simulink model "mcb_pmsm_foc_sensorless_f28379d"  (R2023b)
settings: Solver=FixedStepDiscrete  StartTime=0.0  StopTime=6  FixedStep=Auto  RelTol=1e-3  EnableMultiTasking=on
InitFcn:
  | mcb_pmsm_foc_sensorless_f28379d_datascript;
model workspace (MAT data in the model file):
  encoderResolution = 2000
  hallOffset = '0.5'
  indexOffset = 850
  polePairs = '4'
values from neighbouring files (symbols this model uses):
  acceleration = 0.5/Ts_speed/PU_System.N_base    [mcb_pmsm_foc_sensorless_f28379d_datascript.m]
  dataType = 'single'    [mcb_pmsm_foc_sensorless_f28379d_datascript.m]    (also in mcb_pmsm_foc_test_f28379d_data.m)
  inverter = mcb_updateInverterParameters(pmsm,inverter,target)    [mcb_pmsm_foc_sensorless_f28379d_datascript.m]    (also in mcb_pmsm_foc_test_f28379d_data.m)
  PI_params = mcb_SetControllerParameters(pmsm,inverter,PU_System,T_pwm,2*Ts,Ts_speed)    [mcb_pmsm_foc_sensorless_f28379d_datascript.m]    (also in mcb_pmsm_foc_test_f28379d_data.m = mcb_SetControllerParameters(pmsm,inverter,PU_System,T_pwm,Ts)
  pmsm = mcb_SetPMSMMotorParameters("new")    [mcb_pmsm_foc_sensorless_f28379d_datascript.m]    (also in mcb_pmsm_foc_test_f28379d_data.m = mcb_SetPMSMMotorParameters("SF2804"))
  PU_System = mcb_SetPUSystem(pmsm,inverter)    [mcb_pmsm_foc_sensorless_f28379d_datascript.m]    (also in mcb_pmsm_foc_test_f28379d_data.m)
  Speed_openLoop_PU = 0.1    [mcb_pmsm_foc_sensorless_f28379d_datascript.m]
  T = Ts    (= 5e-05)    [mcb_pmsm_foc_sensorless_f28379d_datascript.m]
  T_Ref_openLoop = 1    [mcb_pmsm_foc_sensorless_f28379d_datascript.m]
  target = mcb_SetProcessorDetails('F28379D',PWM_frequency)    [mcb_pmsm_foc_sensorless_f28379d_datascript.m]    (also in mcb_pmsm_foc_test_f28379d_data.m)
  Ts = T_pwm    [discrete_tansfer_fcn.m]    (also in mcb_pmsm_foc_sensorless_f28379d_datascript.m = 5e-05; mcb_pmsm_foc_test_f28379d_data.m = 5e-05)
  Ts_motor = T_pwm/2    (= 2.5e-05)    [mcb_pmsm_foc_sensorless_f28379d_datascript.m]    (also in mcb_pmsm_foc_test_f28379d_data.m)
  Ts_sensor = 20*Ts    (= 0.001)    [mcb_pmsm_foc_sensorless_f28379d_datascript.m]    (also in mcb_pmsm_foc_test_f28379d_data.m; virtual_speed.m)
  Ts_simulink = T_pwm/2    (= 2.5e-05)    [mcb_pmsm_foc_sensorless_f28379d_datascript.m]    (also in mcb_pmsm_foc_test_f28379d_data.m)
  Ts_speed = 20*Ts    (= 0.001)    [mcb_pmsm_foc_sensorless_f28379d_datascript.m]    (also in mcb_pmsm_foc_test_f28379d_data.m = 0.0005)
undefined symbols (not defined in the file or in its folder): DiscIntNeverNeededParam, Down, GPTRIP1SEL, GPTRIP2SEL, TZ1, TZ2, Up
libraries: mcbcontrolslib x13, simulink x12, c2802xlib x7, mcbpositiondecoderlib x5, c280xlib x5, slpidlib x4, c2837xDlib x4, mcbsensorlessestimatorlib x2, svdschedulerlib x2, svdutilitieslib x1, mcbplantlib x1, autolibpmsmexterior x1
(part 3 of 4)

== system mcb_pmsm_foc_sensorless_f28379d/Current Control/Input Scaling/Calculate position and speed/EKF Observer ==
  InputSignals : Inport
  Action Port : ActionPort  ActionPortLabel=case [ 3 ]:
  Cast To Single : DataTypeConversion  OutDataTypeStr=single  SaturateOnIntegerOverflow=off  RndMeth=Floor
  Data Store Read1 : DataStoreRead  DataStoreName=Enable  IndexOptions=Index vector (dialog)  Indices=1  OutputSizes=1
  Demux1 : Demux
  EKF : Subsystem
  Logical Operator : Logic  Operator=NOT  IconShape=distinctive  AllPortsSameDT=off  OutDataTypeStr=boolean
  Mux2 : Mux  Inputs=2
  Position/Speed : Outport
  wires:
  Data Store Read1/1 -> Logical Operator/1
  InputSignals/1 -> Demux1/1
  Demux1/1 -> EKF/1(ualpha)
  Demux1/2 -> EKF/2(ubeta)
  Demux1/3 -> EKF/3(i_alpha)  "Ialpha"
  Demux1/4 -> EKF/4(i_beta)  "Ibeta"
  Mux2/1 -> Cast To Single/1
  Cast To Single/1 -> Position/Speed/1
  Logical Operator/1 -> EKF/5(Rst)
  EKF/1(theta_hat) -> Mux2/1
  EKF/2(omega_hat) -> Mux2/2  "omega_hat"

== system mcb_pmsm_foc_sensorless_f28379d/Current Control/Input Scaling/Calculate position and speed/Extended EMF Observer ==
  InputSignals : Inport
  Action Port : ActionPort  ActionPortLabel=case [ 2 ]:
  Data Store Read1 : DataStoreRead  DataStoreName=Enable  IndexOptions=Index vector (dialog)  Indices=1  OutputSizes=1
  Demux1 : Demux
  Extended EMF Observer : mcbsensorlessestimatorlib/Extended EMF Observer  InputUnit=Per-unit  PosOut=Electrical position  BlkSampleTime=Ts  StatorResistance=pmsm.Rs  StatorDaxisInductance=pmsm.Ld  StatorQaxisInductance=pmsm.Lq  MaxApplicationSpeed=pmsm.N_base  PolePairs=pmsm.p  MaxStatorVoltage=PU_System.V_base  MaxStatorCurrent=PU_System.I_base  Alpha=10  EEMFCutoffFreq=7500  Kp=250  Ki=200000  N_points=1024  SpeedCutoffFreq=15  PositionUnit=Per-unit  PositionDataType=dataType  SpeedUnit=Per-unit  PerUnitSpeed=PU_System.N_base  SpeedDataType=dataType  TableDatatype=single
      settings: LibrarySourceBlock=mcblib/Sensorless Estimators/Extended EMF Observer
  Logical Operator : Logic  Operator=NOT  IconShape=distinctive  AllPortsSameDT=off  OutDataTypeStr=boolean
  Mux2 : Mux  Inputs=2
  Position/Speed : Outport
  wires:
  Mux2/1 -> Position/Speed/1
  Demux1/3 -> Extended EMF Observer/3  "Ialpha"
  Demux1/4 -> Extended EMF Observer/4  "Ibeta"
  Logical Operator/1 -> Extended EMF Observer/5
  Data Store Read1/1 -> Logical Operator/1
  Demux1/1 -> Extended EMF Observer/1
  Demux1/2 -> Extended EMF Observer/2
  InputSignals/1 -> Demux1/1
  Extended EMF Observer/1 -> Mux2/1
  Extended EMF Observer/2 -> Mux2/2

== system mcb_pmsm_foc_sensorless_f28379d/Current Control/Input Scaling/Calculate position and speed/Flux Observer ==
  InputSignals : Inport
  Action Port : ActionPort  ActionPortLabel=case [ 1 ]:
  DC component removal : Subsystem
  Data Store Read1 : DataStoreRead  DataStoreName=Enable  IndexOptions=Index vector (dialog)  Indices=1  OutputSizes=1
  Demux1 : Demux
  Flux Observer : mcbpositiondecoderlib/Flux Observer  MotorSelection=PMSM  DataTypeSelect=off  BlockInputUnit=Per-unit  PerUnitVoltage=PU_System.V_base  PerUnitCurrent=PU_System.I_base  PositionSelect=on  FluxSelect=off  TorqueSelect=off  PolePairs=4  StatorResistance=pmsm.Rs  StatorDAxisInductance=pmsm.Ld  StatorLeakageInductance=0.0068  RotorLeakageInductance=0.0068  MagnetizingInductance=0.0300  CutoffFreq=3.1863  BlockSampleTime=Ts  PositionUnit=Per-unit  PositionDatatype=dataType  FluxUnit=Weber  PerUnitFlux=0.1  FluxDatatype=single  TorqueUnit=Nm  PerUnitTorque=100  TorqueDatatype=single  DataType=0
  IIR Filter4 : mcbcontrolslib/IIR Filter  VariantControl=Low Pass Filter  VariantSelect=Low-pass  Filter_constant=0.01  advancedSettings=off  Ts=50e-6  cutOff_freq=32.1525
  Logical Operator : Logic  Operator=NOT  IconShape=distinctive  AllPortsSameDT=off  OutDataTypeStr=boolean
  Mux2 : Mux  Inputs=2
  Speed Measurement : mcbpositiondecoderlib/Speed Measurement  PositionUnit=Per unit  PositionScalingDatatype=uint32  SpeedCalculationMode=Time interval for speed calculation  SampleTimeAsync=Ts  MaximumApplicationSpeed=60000  SpeedResolution=5e-6  DelayLength=10  MaximumMeasurableSpeed=59999  MeasurableSpeedResolution=2.794e-05  SpeedUnit=Per unit based on dialog  PerUnitSpeed=PU_System.N_base  SpeedDataType=dataType
  elect2mech : Gain  Gain=1/pmsm.p  RndMeth=Simplest  OutDataTypeStr=Inherit: Same as input
  Position/Speed : Outport
  wires:
  InputSignals/1 -> DC component removal/1(SigIN)
  Mux2/1 -> Position/Speed/1
  Speed Measurement/1 -> IIR Filter4/1
  elect2mech/1 -> Mux2/2
  Demux1/3 -> Flux Observer/3  "Ialpha"
  Demux1/4 -> Flux Observer/4  "Ibeta"
  IIR Filter4/1 -> elect2mech/1
  Logical Operator/1 -> Flux Observer/5
  Data Store Read1/1 -> Logical Operator/1
  Flux Observer/1 -> Mux2/1, Speed Measurement/1
  Demux1/1 -> Flux Observer/1
  Demux1/2 -> Flux Observer/2
  DC component removal/1(SigOUT) -> Demux1/1

== system mcb_pmsm_foc_sensorless_f28379d/Current Control/Input Scaling/Calculate position and speed/HFI ==
  InputSignals : Inport
  Action Port : ActionPort  ActionPortLabel=case [ 4 ]:
  Cast To Single : DataTypeConversion  OutDataTypeStr=single  SaturateOnIntegerOverflow=off  RndMeth=Floor
  Data Store Read1 : DataStoreRead  DataStoreName=Enable  IndexOptions=Index vector (dialog)  Indices=1  OutputSizes=1
  Demux1 : Demux
  Logical Operator : Logic  Operator=NOT  IconShape=distinctive  AllPortsSameDT=off  OutDataTypeStr=boolean
  Mux2 : Mux  Inputs=2
  位置和转速观测器 : Subsystem
  Position/Speed : Outport
  wires:
  Data Store Read1/1 -> Logical Operator/1
  InputSignals/1 -> Demux1/1
  Demux1/3 -> 位置和转速观测器/1(Ialpha)  "Ialpha"
  Demux1/4 -> 位置和转速观测器/2(Ibeta)  "Ibeta"
  Mux2/1 -> Cast To Single/1
  Cast To Single/1 -> Position/Speed/1
  Logical Operator/1 -> ?
  位置和转速观测器/1(theta_est) -> Mux2/1
  位置和转速观测器/2(speed_est) -> Mux2/2  "omega_hat"

== system mcb_pmsm_foc_sensorless_f28379d/Current Control/Input Scaling/Calculate position and speed/Sliding Mode Observer ==
  InputSignals : Inport
  Action Port : ActionPort  ActionPortLabel=case [ 0 ]:
  Data Store Read1 : DataStoreRead  DataStoreName=Enable  IndexOptions=Index vector (dialog)  Indices=1  OutputSizes=1
  Demux1 : Demux
  Logical Operator : Logic  Operator=NOT  IconShape=distinctive  AllPortsSameDT=off  OutDataTypeStr=boolean
  Mux : Mux  Inputs=2
  Sliding Mode Observer : mcbsensorlessestimatorlib/Sliding Mode Observer  InputUnit=Per-unit  BlkSampleTime=Ts  StatorResistance=pmsm.Rs  StatorInductance=pmsm.Ld  MaxApplicationSpeed=pmsm.N_base  PolePairs=pmsm.p  MaxStatorVoltage=PU_System.V_base  MaxStatorCurrent=PU_System.I_base  DisturbanceObserverGain=smo.BackEmfObsGain  CurrentObserverGain=smo.CurrentObsGain  CutoffFreq=smo.CutoffFreq  PositionUnit=Per unit  PositionDataType=dataType  SpeedUnit=Per unit  PerUnitSpeed=PU_System.N_base  SpeedDataType=dataType
  Position/Speed : Outport
  wires:
  Mux/1 -> Position/Speed/1
  Demux1/4 -> Sliding Mode Observer/4  "Ibeta"
  Demux1/3 -> Sliding Mode Observer/3  "Ialpha"
  Sliding Mode Observer/1 -> Mux/1
  InputSignals/1 -> Demux1/1
  Data Store Read1/1 -> Logical Operator/1
  Logical Operator/1 -> Sliding Mode Observer/5
  Sliding Mode Observer/2 -> Mux/2
  Demux1/1 -> Sliding Mode Observer/1
  Demux1/2 -> Sliding Mode Observer/2

== system mcb_pmsm_foc_sensorless_f28379d/Current Control/SCI_Tx/Code Generation/Data_Conditioning_Tx ==
  In1 : Inport
  Data_Type_Fixed_Point : Subsystem  VariantControl=~isequal(dataType,'single')
  Data_Type_Float : Subsystem  VariantControl=isequal(dataType, 'single')
  Data_Log : Outport

== system mcb_pmsm_foc_sensorless_f28379d/Current Control/SCI_Tx/Code Generation/Data_Logging ==
  note: Fast Serial Data Monitoring (32-bit)
  Data_Log : Inport
  Counter Limited : simulink/Sources/Counter Limited  uplimit=600-1  tsamp=-1
  Data : Subsystem  TreatAsAtomicUnit=on
  End : Subsystem  TreatAsAtomicUnit=on
  If : If  IfExpression=u1 == 0  ElseIfExpressions=u1 == 599
  Merge : Merge  Inputs=3
  Merge1 : Merge  Inputs=3
  Mux : Mux  Inputs=2
  Start : Subsystem  TreatAsAtomicUnit=on
  Width : Width  OutDataTypeMode=All ports same datatype  DataType=uint16
  SCI_Tx : Outport
  wires:
  If/3 -> Data/Action
  Data/1(Data_out) -> Merge/3
  Width/1 -> Data/2(Data_width), Start/2(Data_width), End/2(Data_width)
  Merge/1 -> Mux/1  "SCI_Tx_Data"
  Counter Limited/1 -> If/1
  Start/2(Iteration) -> Merge1/1
  Start/1(Data_out) -> Merge/1
  If/2 -> End/Action
  Merge1/1 -> Mux/2  "SCI_Tx_Iteration"
  If/1 -> Start/Action
  End/1(Data_out) -> Merge/2
  End/2(Iteration) -> Merge1/2
  Data/2(Iteration) -> Merge1/3
  Mux/1 -> SCI_Tx/1
  Data_Log/1 -> Width/1, Start/1(Data), End/1(Data), Data/1(Data)

== system mcb_pmsm_foc_sensorless_f28379d/Current Control/SCI_Tx/Code Generation/While Iterator Subsystem ==
  Data : Inport
  Iteration : Inport  Port=2
  Add : Sum  Inputs=+-  OutDataTypeStr=Inherit: Same as first input
  Index Vector : MultiPortSwitch  Inputs=1  SaturateOnIntegerOverflow=off  InputSameDT=off
  SCI Transmit : c280xlib/SCI Transmit  sciModule=A  dataHead=''  dataTail=''  frameSize=1  blockingMode=on  outputStatus=off
  While Iterator : WhileIterator  MaxIters=-1  WhileBlockType=do-while  ShowIterationPort=on  OutputDataType=int16
  wires:
  While Iterator/1 -> Add/2, Index Vector/1
  Data/1 -> Index Vector/2
  Index Vector/1 -> SCI Transmit/1
  Add/1 -> While Iterator/1
  Iteration/1 -> Add/1

== system mcb_pmsm_foc_sensorless_f28379d/Hardware Init/Variant Subsystem/Code Generation/Calculate ADC Offset  ==
  Enable : EnablePort
  Constant : Constant  Value=8
  Constant1 : Constant  Value=inverter.CtSensOffsetMax  OutDataTypeStr=Inherit: Inherit via back propagation
  Constant2 : Constant  Value=inverter.CtSensOffsetMin  OutDataTypeStr=Inherit: Inherit via back propagation
  Divide : Product  Inputs=*/  OutDataTypeStr=uint16
  Divide1 : Product  Inputs=*/  OutDataTypeStr=uint16
  For Iterator Subsystem : Subsystem  TreatAsAtomicUnit=on
  If : If  NumInputs=3  IfExpression=u1 > u3 & u1 < u2
  If Action Subsystem : Subsystem  TreatAsAtomicUnit=on
  If Action Subsystem1 : Subsystem  TreatAsAtomicUnit=on
  If Action Subsystem2 : Subsystem  TreatAsAtomicUnit=on
  If Action Subsystem3 : Subsystem  TreatAsAtomicUnit=on
  If1 : If  NumInputs=3  IfExpression=u1 > u3 & u1 < u2
  wires:
  For Iterator Subsystem/2(Out2) -> Divide1/1
  Divide/1 -> If Action Subsystem/1(In1), If/1
  For Iterator Subsystem/1(Out1) -> Divide/1
  Constant/1 -> Divide1/2, Divide/2
  Divide1/1 -> If Action Subsystem2/1(In1), If1/1
  If/1 -> If Action Subsystem/Action
  If/2 -> If Action Subsystem1/Action
  If1/1 -> If Action Subsystem2/Action
  If1/2 -> If Action Subsystem3/Action
  Constant1/1 -> If1/2, If/2
  Constant2/1 -> If/3, If1/3

== system mcb_pmsm_foc_sensorless_f28379d/Hardware Init/Variant Subsystem/Code Generation/DRV Enable ==
  note: Enable inverter in CPU1
  In : Inport
  ADC Gain Setting : Subsystem
  Constant : Constant  Value=inverter.EnableLogic
  Digital Output : c2837xDlib/Digital Output  Priority=10  GPIO_Number=GPIO120~GPIO127  GPIO_Bit0=off  GPIO_BIT0_Toggle=off  GPIO_Bit1=off  GPIO_BIT1_Toggle=off  GPIO_Bit2=off  GPIO_BIT2_Toggle=off  GPIO_Bit3=off  GPIO_BIT3_Toggle=off  GPIO_Bit4=on  GPIO_BIT4_Toggle=off  GPIO_Bit5=off  GPIO_BIT5_Toggle=off  GPIO_Bit6=off  GPIO_BIT6_Toggle=off  GPIO_Bit7=off  GPIO_BIT7_Toggle=off
  Digital Output1 : c2837xDlib/Digital Output  Priority=10  GPIO_Number=GPIO16~GPIO23  GPIO_Bit0=off  GPIO_BIT0_Toggle=off  GPIO_Bit1=off  GPIO_BIT1_Toggle=off  GPIO_Bit2=off  GPIO_BIT2_Toggle=off  GPIO_Bit3=off  GPIO_BIT3_Toggle=off  GPIO_Bit4=off  GPIO_BIT4_Toggle=off  GPIO_Bit5=off  GPIO_BIT5_Toggle=off  GPIO_Bit6=on  GPIO_BIT6_Toggle=off  GPIO_Bit7=off  GPIO_BIT7_Toggle=off
  Inverter Enable : Constant  OutDataTypeStr=uint16  SampleTime=-1
  NOT : Logic  Operator=NOT  IconShape=distinctive  AllPortsSameDT=off  OutDataTypeStr=boolean
  RunTimeMeasurement : Constant  OutDataTypeStr=uint16  SampleTime=-1
  Switch : Switch  Criteria=u2 > Threshold  SaturateOnIntegerOverflow=off  InputSameDT=off
  wires:
  RunTimeMeasurement/1 -> Digital Output1/1
  NOT/1 -> Switch/3  "Active low logic for inverter enable"
  Inverter Enable/1 -> Switch/1, NOT/1  "Active high logic for inverter enable"
  Constant/1 -> ADC Gain Setting/Enable, Switch/2
  Switch/1 -> Digital Output/1
  In/1 -> ADC Gain Setting/1(In1)

== system mcb_pmsm_foc_sensorless_f28379d/Hardware Init/Variant Subsystem/Code Generation/Default ADC Offset ==
  Enable : EnablePort
  Constant : Constant  Value=inverter.CtSensAOffset  OutDataTypeStr=Inherit: Inherit via back propagation
  Constant1 : Constant  Value=inverter.CtSensBOffset  OutDataTypeStr=Inherit: Inherit via back propagation
  Data Store Write1 : DataStoreWrite  DataStoreName=IaOffset  IndexOptions=Index vector (dialog)  Indices=1  OutputSizes=1
  Data Store Write2 : DataStoreWrite  DataStoreName=IbOffset  IndexOptions=Index vector (dialog)  Indices=1  OutputSizes=1
  wires:
  Constant/1 -> Data Store Write1/1
  Constant1/1 -> Data Store Write2/1

== system mcb_pmsm_foc_sensorless_f28379d/Serial Receive/SCI_Rx/Code Generation/Data_Type_Fixed_Point ==
  SCI Receive : c280xlib/SCI Receive  sciModule=A  dataHead=''  headerCheckMaxCount=16  dataTail=''  dataType=uint32  dataLenOptions=Length via dialog  dataDim=2  maxDataLength=1  initValue=0  errOption=Output the last received value  errValue=0  sampleTime=-1  blockingMode=on  timeOut=0.00875  outputStatus=off
  Data : Outport
  wires:
  SCI Receive/1 -> Data/1

== system mcb_pmsm_foc_sensorless_f28379d/Serial Receive/SCI_Rx/Code Generation/Data_Type_Float ==
  SCI Receive : c280xlib/SCI Receive  sciModule=A  dataHead=''  headerCheckMaxCount=16  dataTail=''  dataType=single  dataLenOptions=Length via dialog  dataDim=2  maxDataLength=1  initValue=0  errOption=Output the last received value  errValue=0  sampleTime=-1  blockingMode=on  timeOut=0.00875  outputStatus=off
  Data : Outport
  wires:
  SCI Receive/1 -> Data/1

== system mcb_pmsm_foc_sensorless_f28379d/Serial Receive/SCI_Rx/Simulation/Data_Conditioning_Tx ==
  In1 : Inport
  In2 : Inport  Port=2
  Data_Type_Fixed_Point : Subsystem  VariantControl=~isequal(dataType, 'single')
  Data_Type_Float : Subsystem  VariantControl=isequal(dataType, 'single')
  Data : Outport

== system mcb_pmsm_foc_sensorless_f28379d/Serial Receive/SCI_Rx/Simulation/Parse ==
  Enable_PWM : Inport
  Debug_signals : Inport  Port=2
  Bitwise Operator : simulink/Logic and Bit Operations/Bitwise Operator  logicop=AND  UseBitMask=on  BitMask=hex2dec('0001')  BitMaskRealWorld=Stored Integer
  Bitwise Operator1 : simulink/Logic and Bit Operations/Bitwise Operator  logicop=AND  UseBitMask=on  BitMask=hex2dec('00F0')  BitMaskRealWorld=Stored Integer
  Shift Arithmetic1 : ArithShift  BitShiftNumber=-4
  Sum : Sum
  Data : Outport
  wires:
  Bitwise Operator/1 -> Sum/1
  Debug_signals/1 -> Shift Arithmetic1/1
  Sum/1 -> Data/1
  Shift Arithmetic1/1 -> Bitwise Operator1/1
  Enable_PWM/1 -> Bitwise Operator/1
  Bitwise Operator1/1 -> Sum/2

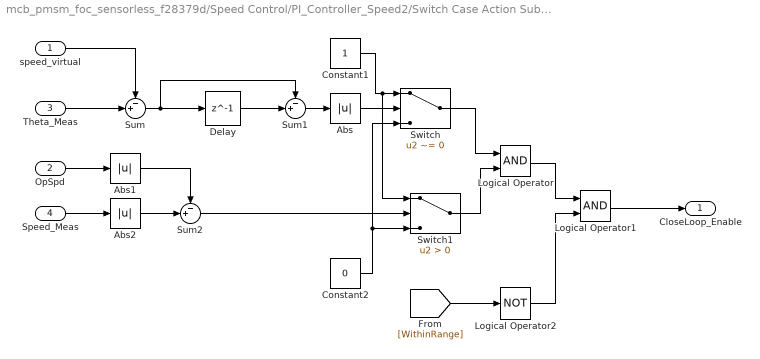
== system mcb_pmsm_foc_sensorless_f28379d/Speed Control/PI_Controller_Speed2/Switch Case Action Subsystem2/Subsystem ==
  speed_virtual : Inport
  OpSpd : Inport  Port=2
  Theta_Meas : Inport  Port=3
  Speed_Meas : Inport  Port=4
  Abs : Abs  SaturateOnIntegerOverflow=off
  Abs1 : Abs  SaturateOnIntegerOverflow=off
  Abs2 : Abs  SaturateOnIntegerOverflow=off
  Constant1 : Constant  OutDataTypeStr=boolean
  Constant2 : Constant  Value=0  OutDataTypeStr=boolean
  Delay : Delay  DelayLength=1  InitialCondition=0
  Logical Operator : Logic  AllPortsSameDT=off  OutDataTypeStr=boolean
  Logical Operator1 : Logic  AllPortsSameDT=off  OutDataTypeStr=boolean
  Logical Operator2 : Logic  Operator=NOT  AllPortsSameDT=off  OutDataTypeStr=boolean
  Sum : Sum  Inputs=-+|
  Sum1 : Sum  Inputs=-+|
  Sum2 : Sum  Inputs=-+|
  Switch : Switch  Criteria=u2 ~= 0  SaturateOnIntegerOverflow=off  InputSameDT=off
  Switch1 : Switch  Criteria=u2 > Threshold  SaturateOnIntegerOverflow=off  InputSameDT=off
  CloseLoop_Enable : Outport
  wires:
  [WithinRange] -> Logical Operator2/1
  Abs/1 -> Switch/2
  Sum2/1 -> Switch1/2
  Constant1/1 -> Switch1/1, Switch/1
  Constant2/1 -> Switch/3, Switch1/3
  Abs1/1 -> Sum2/1
  Logical Operator2/1 -> Logical Operator1/2
  Switch1/1 -> Logical Operator/2
  Sum/1 -> Sum1/1, Delay/1
  Logical Operator/1 -> Logical Operator1/1
  Abs2/1 -> Sum2/2
  Sum1/1 -> Abs/1
  Switch/1 -> Logical Operator/1
  Delay/1 -> Sum1/2
  OpSpd/1 -> Abs1/1
  speed_virtual/1 -> Sum/1
  Logical Operator1/1 -> CloseLoop_Enable/1
  Speed_Meas/1 -> Abs2/1
  Theta_Meas/1 -> Sum/2

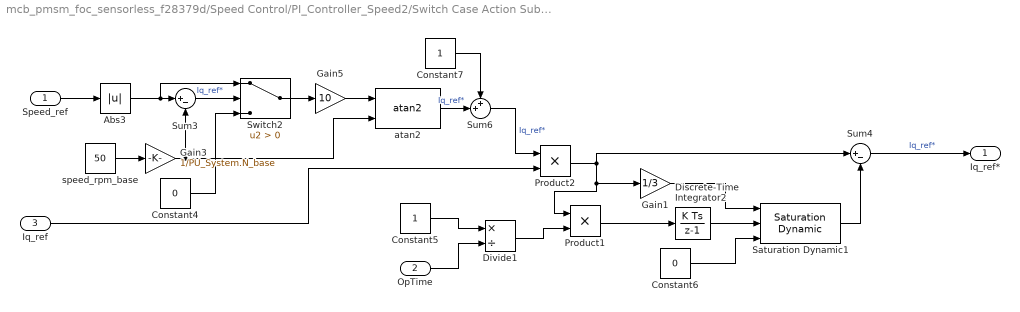
== system mcb_pmsm_foc_sensorless_f28379d/Speed Control/PI_Controller_Speed2/Switch Case Action Subsystem2/Subsystem1 ==
  Speed_ref : Inport
  OpTime : Inport  Port=2
  Iq_ref : Inport  Port=3
  Abs3 : Abs  SaturateOnIntegerOverflow=off
  Constant4 : Constant  Value=0
  Constant5 : Constant
  Constant6 : Constant  Value=0
  Constant7 : Constant
  Discrete-Time Integrator2 : DiscreteIntegrator  SampleTime=-1  OutDataTypeStr=single  ICPrevOutput=DiscIntNeverNeededParam  ICPrevScaledInput=DiscIntNeverNeededParam
  Divide1 : Product  Inputs=*/
  Gain1 : Gain  Gain=1/3
  Gain3 : Gain  Gain=1/PU_System.N_base
  Gain5 : Gain  Gain=10
  Product1 : Product  OutDataTypeStr=single
  Product2 : Product  OutDataTypeStr=single
  Saturation Dynamic1 : simulink/Discontinuities/Saturation Dynamic  OutMin=[]  OutMax=[]  OutDataTypeStr=single  OutDataType=fixdt(1, 16)  OutScaling=2^-10  DoSatur=off
  Sum3 : Sum  Inputs=|+-
  Sum4 : Sum  Inputs=|+-
  Sum6 : Sum  Inputs=++|
  Switch2 : Switch  Criteria=u2 > Threshold  SaturateOnIntegerOverflow=off  InputSameDT=off
  atan2 : mcbcontrolslib/atan2  ApproximationMethod=None  NumberOfIterations=11  NumberOfDataPoints=16  InterpMethod=Flat  outputUnit=PerUnit  TableDataTypeStr=Inherit: Inherit via input
      settings: LibrarySourceBlock=mcblib/Controls/Math Transforms/atan2
  speed_rpm_base : Constant  Value=50
  Iq_ref* : Outport
  wires:
  Sum6/1 -> Product2/1  "Iq_ref*"
  Gain1/1 -> Saturation Dynamic1/1
  Abs3/1 -> Switch2/1, Sum3/1
  Product2/1 -> Sum4/1, Gain1/1, Product1/1
  Gain3/1 -> atan2/2, Sum3/2
  Sum3/1 -> Switch2/2  "Iq_ref*"
  Discrete-Time Integrator2/1 -> Saturation Dynamic1/2
  Gain5/1 -> atan2/1
  OpTime/1 -> Divide1/2
  Divide1/1 -> Product1/2
  Iq_ref/1 -> Product2/2
  Switch2/1 -> Gain5/1
  Sum4/1 -> Iq_ref*/1  "Iq_ref*"
  speed_rpm_base/1 -> Gain3/1
  Constant4/1 -> Switch2/3
  Constant7/1 -> Sum6/1
  Saturation Dynamic1/1 -> Sum4/2
  Constant5/1 -> Divide1/1
  Product1/1 -> Discrete-Time Integrator2/1
  Constant6/1 -> Saturation Dynamic1/3
  atan2/1 -> Sum6/2  "Iq_ref*"
  Speed_ref/1 -> Abs3/1

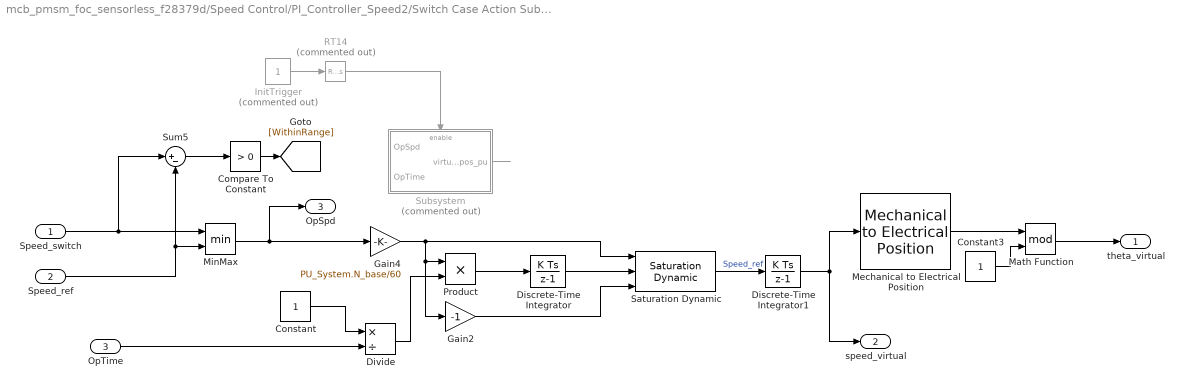
== system mcb_pmsm_foc_sensorless_f28379d/Speed Control/PI_Controller_Speed2/Switch Case Action Subsystem2/Subsystem2 ==
  Speed_switch : Inport
  Speed_ref : Inport  Port=2
  OpTime : Inport  Port=3
  Compare To Constant : simulink/Logic and Bit Operations/Compare To Constant  relop=>  const=0  OutDataTypeStr=boolean
  Constant : Constant
  Constant3 : Constant  OutDataTypeStr=single
  Discrete-Time Integrator : DiscreteIntegrator  SampleTime=-1  OutDataTypeStr=single  ICPrevOutput=DiscIntNeverNeededParam  ICPrevScaledInput=DiscIntNeverNeededParam
  Discrete-Time Integrator1 : DiscreteIntegrator  SampleTime=-1  OutDataTypeStr=single  ICPrevOutput=DiscIntNeverNeededParam  ICPrevScaledInput=DiscIntNeverNeededParam
  Divide : Product  Inputs=*/
  Gain2 : Gain  Gain=-1
  Gain4 : Gain  Gain=PU_System.N_base/60
  InitTrigger : Constant  Priority=10  Commented=on  OutDataTypeStr=boolean
  Math Function : Math  Operator=mod
  Mechanical to Electrical Position : mcbpositiondecoderlib/Mechanical to Electrical Position  PolePairsInputType=Specify via dialog  NrPP=pmsm.p  selectedRange=Per unit  MechOfstInputType=Specify via dialog  mechOffsetIn=0  maxAngleIn=1  InputDataType=dataType  VariantSelect=floating-point
  MinMax : MinMax  Inputs=2
  Product : Product  OutDataTypeStr=single
  RT14 : RateTransition  Commented=on  Deterministic=off  OutPortSampleTime=Ts_sensor
  Saturation Dynamic : simulink/Discontinuities/Saturation Dynamic  OutMin=[]  OutMax=[]  OutDataTypeStr=single  OutDataType=fixdt(1, 16)  OutScaling=2^-10  DoSatur=off
  Subsystem : Subsystem  Commented=on
  Sum5 : Sum  Inputs=|+-
  theta_virtual : Outport
  speed_virtual : Outport  Port=2
  OpSpd : Outport  Port=3
  wires:
  Gain4/1 -> Saturation Dynamic/1, Gain2/1, Product/1
  Saturation Dynamic/1 -> Discrete-Time Integrator1/1  "Speed_ref"
  Gain2/1 -> Saturation Dynamic/3
  MinMax/1 -> OpSpd/1, Gain4/1
  Discrete-Time Integrator/1 -> Saturation Dynamic/2
  Speed_switch/1 -> Sum5/1, MinMax/1
  Speed_ref/1 -> Sum5/2, MinMax/2
  Compare To Constant/1 -> [WithinRange]
  OpTime/1 -> Divide/2
  InitTrigger/1 -> RT14/1
  Sum5/1 -> Compare To Constant/1
  Constant/1 -> Divide/1
  Constant3/1 -> Math Function/2
  Product/1 -> Discrete-Time Integrator/1
  Discrete-Time Integrator1/1 -> speed_virtual/1, Mechanical to Electrical Position/1
  Mechanical to Electrical Position/1 -> Math Function/1
  RT14/1 -> Subsystem/Enable
  Divide/1 -> Product/2
  Subsystem/1(virtual_pos_pu) -> ?
  Math Function/1 -> theta_virtual/1

== system mcb_pmsm_foc_sensorless_f28379d/Current Control/Closed Loop/Current_Controllers/Subsystem/Subsystem ==
  Constant : Constant  Value=2
  Data Store Write : DataStoreWrite  DataStoreName=Udh  IndexOptions=Index vector (dialog)  Indices=1  OutputSizes=1
  Delay : Delay  DelayLength=1  InitialCondition=0
  Discrete Pulse Generator : DiscretePulseGenerator  Amplitude=4  SampleTime=-1
  Gain : Gain  Gain=-1
  Subtract : Sum  Inputs=+-
  Unit Delay : UnitDelay  InitialCondition=2  SampleTime=-1  HasFrameUpgradeWarning=on
  Udh : Outport
  wires:
  Unit Delay/1 -> Gain/1
  Gain/1 -> Unit Delay/1
  Subtract/1 -> Data Store Write/1, Udh/1
  Constant/1 -> Subtract/2
  Discrete Pulse Generator/1 -> Subtract/1

== system mcb_pmsm_foc_sensorless_f28379d/Current Control/Input Scaling/Calculate Phase Currents/Data_Type/Data_Type_Fixed_Point ==
  In1 : Inport
  Data Type Conversion : DataTypeConversion  OutDataTypeStr=fixdt(1,32,17)  ConvertRealWorld=Stored Integer (SI)  RndMeth=Simplest  SaturateOnIntegerOverflow=off
  Data Type Conversion1 : DataTypeConversion  OutDataTypeStr=dataType  RndMeth=Simplest  SaturateOnIntegerOverflow=off
  Q17 per unit conversion : ArithShift  BitShiftNumber=-6
  Iab_meas_PU : Outport
  wires:
  In1/1 -> Q17 per unit conversion/1
  Data Type Conversion1/1 -> Iab_meas_PU/1
  Data Type Conversion/1 -> Data Type Conversion1/1
  Q17 per unit conversion/1 -> Data Type Conversion/1

== system mcb_pmsm_foc_sensorless_f28379d/Current Control/Input Scaling/Calculate Phase Currents/Data_Type/Data_Type_Float ==
  In1 : Inport
  Get ADC Voltage : Gain  Gain=target.ADC_Vref /target.ADC_MaxCount  OutDataTypeStr=dataType  RndMeth=Simplest
  Get Currents : Gain  Gain=1/inverter.ISenseVoltPerAmp  RndMeth=Simplest  OutDataTypeStr=Inherit: Same as input
  PU_Conversion : Gain  Gain=1/PU_System.I_base  RndMeth=Simplest  OutDataTypeStr=Inherit: Same as input
  Iab_meas_PU : Outport
  wires:
  Get ADC Voltage/1 -> Get Currents/1
  Get Currents/1 -> PU_Conversion/1
  PU_Conversion/1 -> Iab_meas_PU/1
  In1/1 -> Get ADC Voltage/1

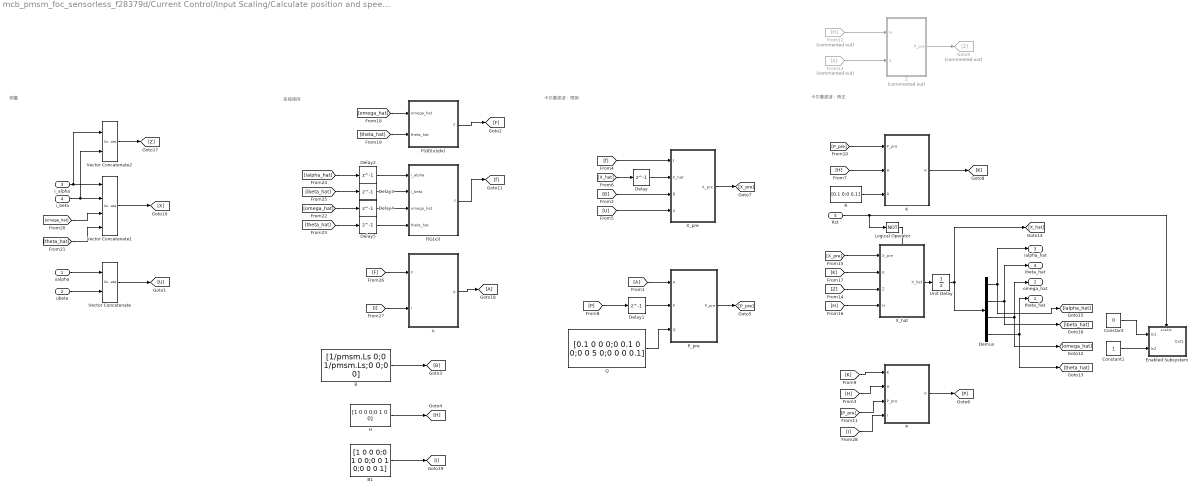
== system mcb_pmsm_foc_sensorless_f28379d/Current Control/Input Scaling/Calculate position and speed/EKF Observer/EKF ==
  note: 卡尔曼滤波：矫正
  note: 测量
  note: 卡尔曼滤波：预测
  note: 系统矩阵
  ualpha : Inport
  ubeta : Inport  Port=2
  i_alpha : Inport  Port=3
  i_beta : Inport  Port=4
  Rst : Inport  Port=5
  A : Subsystem
  B : Constant  Value=[1/pmsm.Ls 0;0 1/pmsm.Ls;0 0;0 0]
  B1 : Constant  Value=[1 0 0 0;0 1 0 0;0 0 1 0;0 0 0 1]
  Constant : Constant  Value=0
  Constant1 : Constant
  Delay{,1..5} (6 alike) : Delay  DelayLength=1  InitialCondition=0
  Demux : Demux
  Enabled Subsystem : Subsystem  TreatAsAtomicUnit=on
  F(dG(x)/dx) : Subsystem
  From1 : From
  From12 : From  Commented=on  GotoTag=H
  From13 : From  Commented=on  GotoTag=X
  Goto18 : Goto
  Goto9 : Goto  Commented=on  GotoTag=Z
  H : Constant  Value=[1 0 0 0;0 1 0 0]
  K : Subsystem
  Logical Operator : Logic  Operator=NOT  IconShape=distinctive  AllPortsSameDT=off  OutDataTypeStr=boolean
  P : Subsystem
  P_pre : Subsystem
  Q : Constant  Value=[0.1 0 0 0;0 0.1 0 0;0 0 5 0;0 0 0 0.1]
  R : Constant  Value=[0.1 0;0 0.1]
  Unit Delay : UnitDelay  InitialCondition=[0;0;0.1;0]  SampleTime=-1  HasFrameUpgradeWarning=on
  Vector Concatenate : Concatenate  Mode=Multidimensional array
  Vector Concatenate1 : Concatenate  NumInputs=4  Mode=Multidimensional array
  Vector Concatenate2 : Concatenate  Mode=Multidimensional array
  X_hat : Subsystem
  X_pre : Subsystem
  Z : Subsystem  Commented=on
  f(G(x)) : Subsystem
  theta_hat : Outport
  omega_hat : Outport  Port=2
  ialpha_hat : Outport  Port=3
  ibeta_hat : Outport  Port=4
  wires:
  Q/1 -> P_pre/3(Q)
  ualpha/1 -> Vector Concatenate/1
  Vector Concatenate/1 -> [U]
  From1/1 -> P_pre/1(A)
  P/1(P) -> [P]
  F(dG(x)/dx)/1(F) -> [F]
  [K] -> P/1(K)
  [P] -> Delay1/1
  [X_pre] -> X_hat/1(X_pre)
  Z/1(P_pre) -> Goto9/1
  Demux/1 -> [ialpha_hat], ialpha_hat/1
  [K] -> X_hat/2(K)
  Demux/2 -> [ibeta_hat], ibeta_hat/1
  [H] -> P/2(H)
  [H] -> K/2(H)
  K/1(K) -> [K]
  From12/1 -> Z/1(H)
  H/1 -> [H]
  B/1 -> [B]
  ubeta/1 -> Vector Concatenate/2
  [X_hat] -> Delay/1
  [B] -> X_pre/3(B)
  [H] -> X_hat/4(H)
  Delay/1 -> X_pre/2(X_hat)
  [P_pre] -> P/3(P_pre)
  R/1 -> K/3(R)
  P_pre/1(P_pre) -> [P_pre]
  [P_pre] -> K/1(P_pre)
  Delay1/1 -> P_pre/2(P)
  [f] -> X_pre/1(f)
  From13/1 -> Z/2(X)
  [omega_hat] -> F(dG(x)/dx)/1(omega_hat)
  X_pre/1(X_pre) -> [X_pre]
  [Z] -> X_hat/3(Z)
  [theta_hat] -> F(dG(x)/dx)/2(theta_hat)
  i_alpha/1 -> Vector Concatenate2/1, Vector Concatenate1/1
  i_beta/1 -> Vector Concatenate2/2, Vector Concatenate1/2
  Vector Concatenate1/1 -> [X]
  [omega_hat] -> Vector Concatenate1/3
  [theta_hat] -> Vector Concatenate1/4
  [U] -> X_pre/4(U)
  f(G(x))/1(f) -> [f]
  [ialpha_hat] -> Delay2/1
  Delay2/1 -> f(G(x))/1(i_alpha)
  [ibeta_hat] -> Delay3/1
  Delay3/1 -> f(G(x))/2(i_beta)
  [omega_hat] -> Delay4/1
  Delay4/1 -> f(G(x))/3(omega_hat)
  [theta_hat] -> Delay5/1
  Delay5/1 -> f(G(x))/4(theta_hat)
  Vector Concatenate2/1 -> [Z]
  [F] -> A/1(F)
  A/1(A) -> Goto18/1
  B1/1 -> [I]
  [I] -> A/2(I)
  [I] -> P/4(I)
  Constant1/1 -> Enabled Subsystem/2(In2)
  Constant/1 -> Enabled Subsystem/1(In1)
  Demux/3 -> [omega_hat], omega_hat/1
  Demux/4 -> [theta_hat], theta_hat/1
  Logical Operator/1 -> ?
  Rst/1 -> Logical Operator/1, Enabled Subsystem/Enable
  X_hat/1(X_hat) -> Unit Delay/1
  Unit Delay/1 -> Demux/1, [X_hat]

== system mcb_pmsm_foc_sensorless_f28379d/Current Control/Input Scaling/Calculate position and speed/Flux Observer/DC component removal ==
  SigIN : Inport
  IIR Filter : mcbcontrolslib/IIR Filter  VariantControl=Low Pass Filter  VariantSelect=Low-pass  Filter_constant=0.005*(Ts/50e-6)  advancedSettings=off  Ts=50e-6  cutOff_freq=15.9955
  Sum6 : Sum  Inputs=|+-  RndMeth=Simplest  OutDataTypeStr=Inherit: Same as first input
  SigOUT : Outport
  wires:
  IIR Filter/1 -> Sum6/2
  SigIN/1 -> IIR Filter/1, Sum6/1
  Sum6/1 -> SigOUT/1

== system mcb_pmsm_foc_sensorless_f28379d/Current Control/Input Scaling/Calculate position and speed/HFI/位置和转速观测器 ==
  Ialpha : Inport
  Ibeta : Inport  Port=2
  Data Store Read1 : DataStoreRead  DataStoreName=Udh  IndexOptions=Index vector (dialog)  Indices=1  OutputSizes=1
  两相静止坐标系提取高频信号 : Subsystem
  位置估算 : Subsystem
  theta_est : Outport
  speed_est : Outport  Port=2
  wires:
  Ialpha/1 -> 两相静止坐标系提取高频信号/1(i_alpha)
  Ibeta/1 -> 两相静止坐标系提取高频信号/2(i_beta)
  两相静止坐标系提取高频信号/1(i_alpha_h) -> 位置估算/1(Ialpha_h)
  两相静止坐标系提取高频信号/2(i_beta_h) -> 位置估算/2(Ibeta_h)
  位置估算/1(Speed_Est) -> speed_est/1
  位置估算/2(theta_e^) -> theta_est/1
  Data Store Read1/1 -> 位置估算/3(Udh)

== system mcb_pmsm_foc_sensorless_f28379d/Current Control/SCI_Tx/Code Generation/Data_Conditioning_Tx/Data_Type_Fixed_Point ==
  In1 : Inport
  Data Type Conversion : DataTypeConversion  OutDataTypeStr=fixdt(1,32,28)  RndMeth=Simplest  SaturateOnIntegerOverflow=off
  Data Type Conversion3 : DataTypeConversion  OutDataTypeStr=uint32  ConvertRealWorld=Stored Integer (SI)  RndMeth=Simplest  SaturateOnIntegerOverflow=off
  Data_Log : Outport
  wires:
  In1/1 -> Data Type Conversion/1
  Data Type Conversion3/1 -> Data_Log/1
  Data Type Conversion/1 -> Data Type Conversion3/1

== system mcb_pmsm_foc_sensorless_f28379d/Current Control/SCI_Tx/Code Generation/Data_Conditioning_Tx/Data_Type_Float ==
  In1 : Inport
  Byte Pack : svdutilitieslib/Byte Pack  maskPackedDataType=uint32  datatypes={'single'}  byteAlign=4  blockPlatform=tic2000
  Data_Log : Outport
  wires:
  Byte Pack/1 -> Data_Log/1
  In1/1 -> Byte Pack/1

== system mcb_pmsm_foc_sensorless_f28379d/Current Control/SCI_Tx/Code Generation/Data_Logging/Data ==
  Data : Inport
  Data_width : Inport  Port=2
  Action Port : ActionPort  ActionPortLabel=else
  Dummy : Constant  Value=hex2dec('0000')  OutDataTypeStr=uint32
  Mux : Mux  Inputs=2
  Data_out : Outport  VectorParamsAs1DForOutWhenUnconnected=off
  Iteration : Outport  Port=2  VectorParamsAs1DForOutWhenUnconnected=off
  wires:
  Data_width/1 -> Iteration/1
  Data/1 -> Mux/1
  Dummy/1 -> Mux/2
  Mux/1 -> Data_out/1

== system mcb_pmsm_foc_sensorless_f28379d/Current Control/SCI_Tx/Code Generation/Data_Logging/End ==
  Data : Inport
  Data_width : Inport  Port=2
  Action Port : ActionPort  ActionPortLabel=elseif(u1 == 599)
  Bias : Bias  Bias=1  SaturateOnIntegerOverflow=off
  End : Constant  Value=hex2dec('45454545')  OutDataTypeStr=uint32
  Mux : Mux  Inputs=2
  Data_out : Outport  VectorParamsAs1DForOutWhenUnconnected=off
  Iteration : Outport  Port=2  VectorParamsAs1DForOutWhenUnconnected=off
  wires:
  Data/1 -> Mux/1
  Data_width/1 -> Bias/1
  Bias/1 -> Iteration/1
  End/1 -> Mux/2
  Mux/1 -> Data_out/1

== system mcb_pmsm_foc_sensorless_f28379d/Current Control/SCI_Tx/Code Generation/Data_Logging/Start ==
  Data : Inport
  Data_width : Inport  Port=2
  Action Port : ActionPort  ActionPortLabel=if(u1 == 0)
  Bias : Bias  Bias=1  SaturateOnIntegerOverflow=off
  Mux : Mux  Inputs=2
  Start : Constant  Value=hex2dec('53535353')  OutDataTypeStr=uint32
  Data_out : Outport  VectorParamsAs1DForOutWhenUnconnected=off
  Iteration : Outport  Port=2  VectorParamsAs1DForOutWhenUnconnected=off
  wires:
  Data/1 -> Mux/2
  Data_width/1 -> Bias/1
  Bias/1 -> Iteration/1
  Start/1 -> Mux/1
  Mux/1 -> Data_out/1

== system mcb_pmsm_foc_sensorless_f28379d/Hardware Init/Variant Subsystem/Code Generation/Calculate ADC Offset /For Iterator Subsystem ==
  ADC_B2 : c2802xlib/ADC  Priority=20  blkParamProc=C2000_Type4  ADCModule=B  samplingMode=Single sample mode  ADCResolution=12-bit (Single-ended input)  useSOC1=SOC2  useSOC2=SOC0_SOC1  SOCAcquisitionWindow=15  SOCTriggerSource=Software  SOCInterruptTrigger=No ADCINT  Ts=-1  dType=uint16  postInterrupt=off  interruptSel=ADCINT1  ADCINTContinuous=on  endma=off  chdma=1  conv1=ADCINA0  conv2=ADCINA0 and ADCINB0  conv1_Type4=ADCIN2  conv2_Type4=ADCIN0 and ADCIN1
  ADC_C2 : c2802xlib/ADC  Priority=20  blkParamProc=C2000_Type4  ADCModule=C  samplingMode=Single sample mode  ADCResolution=12-bit (Single-ended input)  useSOC1=SOC2  useSOC2=SOC0_SOC1  SOCAcquisitionWindow=15  SOCTriggerSource=Software  SOCInterruptTrigger=No ADCINT  Ts=-1  dType=uint16  postInterrupt=off  interruptSel=ADCINT1  ADCINTContinuous=on  endma=off  chdma=1  conv1=ADCINA0  conv2=ADCINA0 and ADCINB0  conv1_Type4=ADCIN2  conv2_Type4=ADCIN0 and ADCIN1
  For Iterator : ForIterator  IterationLimit=16  IterationVariableDataType=uint16
  If : If  IfExpression=u1 > 8  ShowElse=off
  If Action Subsystem : Subsystem  TreatAsAtomicUnit=on
  Out1 : Outport
  Out2 : Outport  Port=2
  wires:
  For Iterator/1 -> If/1
  ADC_C2/1 -> If Action Subsystem/1(In1)
  ADC_B2/1 -> If Action Subsystem/2(In2)
  If Action Subsystem/1(Out1) -> Out1/1
  If Action Subsystem/2(Out2) -> Out2/1
  If/1 -> If Action Subsystem/Action

== system mcb_pmsm_foc_sensorless_f28379d/Hardware Init/Variant Subsystem/Code Generation/Calculate ADC Offset /If Action Subsystem ==
  In1 : Inport
  Action Port : ActionPort  ActionPortLabel=if(u1 > u3 & u1 < u2)
  Data Store Write1 : DataStoreWrite  DataStoreName=IaOffset  IndexOptions=Index vector (dialog)  Indices=1  OutputSizes=1
  wires:
  In1/1 -> Data Store Write1/1

== system mcb_pmsm_foc_sensorless_f28379d/Hardware Init/Variant Subsystem/Code Generation/Calculate ADC Offset /If Action Subsystem1 ==
  Action Port : ActionPort  ActionPortLabel=else
  Constant : Constant  Value=inverter.CtSensAOffset  OutDataTypeStr=Inherit: Inherit via back propagation
  Data Store Write1 : DataStoreWrite  DataStoreName=IaOffset  IndexOptions=Index vector (dialog)  Indices=1  OutputSizes=1
  wires:
  Constant/1 -> Data Store Write1/1

== system mcb_pmsm_foc_sensorless_f28379d/Hardware Init/Variant Subsystem/Code Generation/Calculate ADC Offset /If Action Subsystem2 ==
  In1 : Inport
  Action Port : ActionPort  ActionPortLabel=if(u1 > u3 & u1 < u2)
  Data Store Write2 : DataStoreWrite  DataStoreName=IbOffset  IndexOptions=Index vector (dialog)  Indices=1  OutputSizes=1
  wires:
  In1/1 -> Data Store Write2/1

== system mcb_pmsm_foc_sensorless_f28379d/Hardware Init/Variant Subsystem/Code Generation/Calculate ADC Offset /If Action Subsystem3 ==
  Action Port : ActionPort  ActionPortLabel=else
  Constant1 : Constant  Value=inverter.CtSensBOffset  OutDataTypeStr=Inherit: Inherit via back propagation
  Data Store Write2 : DataStoreWrite  DataStoreName=IbOffset  IndexOptions=Index vector (dialog)  Indices=1  OutputSizes=1
  wires:
  Constant1/1 -> Data Store Write2/1

== system mcb_pmsm_foc_sensorless_f28379d/Hardware Init/Variant Subsystem/Code Generation/DRV Enable/ADC Gain Setting ==
  In1 : Inport
  Enable : EnablePort
  Demux : Demux  Outputs=2
  Display : Display
      settings: Format=hex (Stored Integer)
  Display1 : Display
      settings: Format=hex (Stored Integer)
  SPI Master Transfer : c280xlib/SPI Controller Transfer  SPISelect=SPI_A  ClockPolarity=Rising_edge  ClockPhase=No_delay  SPIModule=uint32(0)  Mode=Master  BusSpeed=uint32(1000000)  FirstBitToTransfer=Most significant bit (MSB)  ClockMode=0  BlockFunction=Transfer  EnableRegisterAddress=off  RegisterAddress=0  OutputDataType=int8  OutputDataLength=1  DataBits=16  UseCustomSSPin=Provided by the SPI peripheral  ActiveLowSSPin=Active low  Pin=61
  SPI Master Transfer1 : c280xlib/SPI Controller Transfer  SPISelect=SPI_A  ClockPolarity=Rising_edge  ClockPhase=No_delay  SPIModule=uint32(0)  Mode=Master  BusSpeed=uint32(1000000)  FirstBitToTransfer=Most significant bit (MSB)  ClockMode=0  BlockFunction=Transfer  EnableRegisterAddress=off  RegisterAddress=0  OutputDataType=int8  OutputDataLength=1  DataBits=16  UseCustomSSPin=Provided by the SPI peripheral  ActiveLowSSPin=Active low  Pin=61
  wires:
  Demux/2 -> SPI Master Transfer1/1
  SPI Master Transfer/1 -> Display/1
  SPI Master Transfer1/1 -> Display1/1
  Demux/1 -> SPI Master Transfer/1
  In1/1 -> Demux/1

== system mcb_pmsm_foc_sensorless_f28379d/Serial Receive/SCI_Rx/Simulation/Data_Conditioning_Tx/Data_Type_Fixed_Point ==
  In1 : Inport
  In2 : Inport  Port=2
  Data Type Conversion : DataTypeConversion  OutDataTypeStr=fixdt(1,32,28)  RndMeth=Simplest  SaturateOnIntegerOverflow=off
  Data Type Conversion1 : DataTypeConversion  OutDataTypeStr=uint32  RndMeth=Simplest  SaturateOnIntegerOverflow=off
  Data Type Conversion3 : DataTypeConversion  OutDataTypeStr=uint32  ConvertRealWorld=Stored Integer (SI)  RndMeth=Simplest  SaturateOnIntegerOverflow=off
  Mux : Mux  Inputs=2
  Data : Outport
  wires:
  In1/1 -> Data Type Conversion/1
  Data Type Conversion3/1 -> Mux/1
  Data Type Conversion/1 -> Data Type Conversion3/1
  In2/1 -> Data Type Conversion1/1
  Data Type Conversion1/1 -> Mux/2
  Mux/1 -> Data/1

== system mcb_pmsm_foc_sensorless_f28379d/Serial Receive/SCI_Rx/Simulation/Data_Conditioning_Tx/Data_Type_Float ==
  In1 : Inport
  In2 : Inport  Port=2
  Data Type Conversion2 : DataTypeConversion  OutDataTypeStr=single  RndMeth=Simplest  SaturateOnIntegerOverflow=off
  Mux : Mux  Inputs=2
  Data : Outport
  wires:
  In1/1 -> Mux/1
  Mux/1 -> Data/1
  In2/1 -> Data Type Conversion2/1
  Data Type Conversion2/1 -> Mux/2

== system mcb_pmsm_foc_sensorless_f28379d/Speed Control/PI_Controller_Speed2/Switch Case Action Subsystem2/Subsystem2/Subsystem ==
  OpSpd : Inport
  OpTime : Inport  Port=2
  Enable : EnablePort
  Constant : Constant  Value=0
  Gain : Gain  Gain=1/Ts_speed
  MATLAB Function : MATLAB Function  TreatAsAtomicUnit=on
  Product : Product
  Saturation Dynamic : simulink/Discontinuities/Saturation Dynamic  OutMin=[]  OutMax=[]  OutDataTypeStr=Inherit: Same as second input  OutDataType=fixdt(1, 16)  OutScaling=2^-10  DoSatur=off
  Ts_sensor : Constant  Value=Ts_sensor
  virtual_pos_pu : Outport
  wires:
  MATLAB Function/1(pu) -> virtual_pos_pu/1
  Ts_sensor/1 -> MATLAB Function/2(Ts)
  Constant/1 -> Saturation Dynamic/3
  Product/1 -> Saturation Dynamic/2
  OpSpd/1 -> Saturation Dynamic/1, Product/1
  Saturation Dynamic/1 -> MATLAB Function/1(speed_ref_rpm)
  Gain/1 -> Product/2
  OpTime/1 -> Gain/1

== system mcb_pmsm_foc_sensorless_f28379d/Current Control/Input Scaling/Calculate position and speed/EKF Observer/EKF/A ==
  F : Inport
  I : Inport  Port=2
  Add1 : Sum
  Constant : Constant
  Gain : Gain  Gain=T
  Matrix Multiply : Product
  A : Outport
  wires:
  F/1 -> Matrix Multiply/1
  I/1 -> Add1/1
  Constant/1 -> Gain/1
  Gain/1 -> Matrix Multiply/2
  Matrix Multiply/1 -> Add1/2
  Add1/1 -> A/1

== system mcb_pmsm_foc_sensorless_f28379d/Current Control/Input Scaling/Calculate position and speed/EKF Observer/EKF/Enabled Subsystem ==
  In1 : Inport
  In2 : Inport  Port=2
  Enable : EnablePort
  Mux : Mux  Inputs=2
  Out1 : Outport
  wires:
  In2/1 -> Mux/2
  Mux/1 -> Out1/1
  In1/1 -> Mux/1

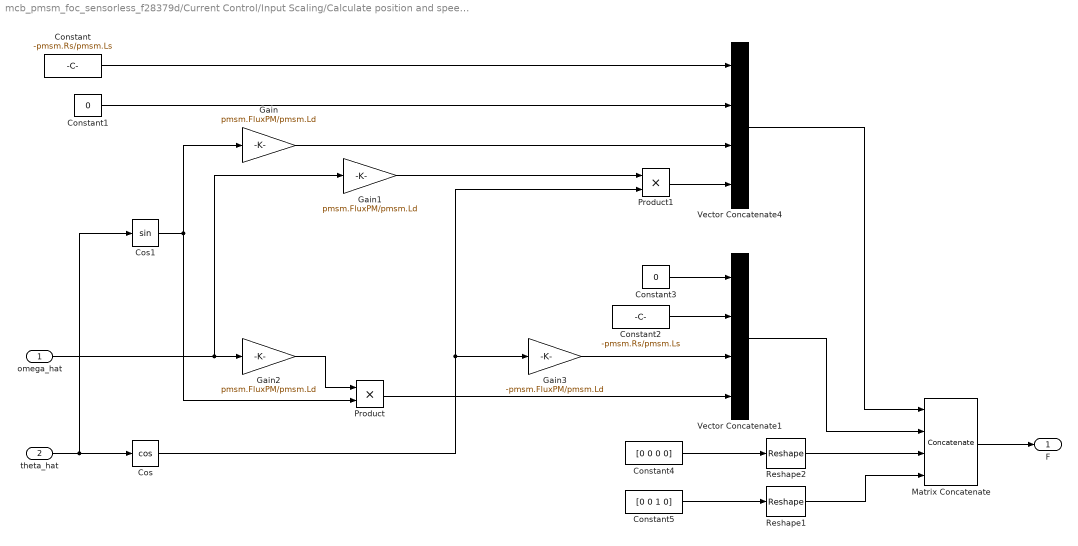
== system mcb_pmsm_foc_sensorless_f28379d/Current Control/Input Scaling/Calculate position and speed/EKF Observer/EKF/F(dG(x)//dx) ==
  omega_hat : Inport
  theta_hat : Inport  Port=2
  Constant : Constant  Value=-pmsm.Rs/pmsm.Ls
  Constant1 : Constant  Value=0
  Constant2 : Constant  Value=-pmsm.Rs/pmsm.Ls
  Constant3 : Constant  Value=0
  Constant4 : Constant  Value=[0 0 0 0]
  Constant5 : Constant  Value=[0 0 1 0]
  Cos : Trigonometry  Operator=cos
  Cos1 : Trigonometry
  Gain : Gain  Gain=pmsm.FluxPM/pmsm.Ld
  Gain1 : Gain  Gain=pmsm.FluxPM/pmsm.Ld
  Gain2 : Gain  Gain=pmsm.FluxPM/pmsm.Ld
  Gain3 : Gain  Gain=-pmsm.FluxPM/pmsm.Ld
  Matrix Concatenate : Concatenate  NumInputs=4  Mode=Multidimensional array
  Product : Product
  Product1 : Product
  Reshape1 : Reshape  OutputDimensionality=Row vector (2-D)
  Reshape2 : Reshape  OutputDimensionality=Row vector (2-D)
  Vector Concatenate1 : Concatenate  NumInputs=4  Mode=Multidimensional array  ConcatenateDimension=2
  Vector Concatenate4 : Concatenate  NumInputs=4  Mode=Multidimensional array  ConcatenateDimension=2
  F : Outport
  wires:
  Vector Concatenate4/1 -> Matrix Concatenate/1
  Vector Concatenate1/1 -> Matrix Concatenate/2
  Constant/1 -> Vector Concatenate4/1
  Constant1/1 -> Vector Concatenate4/2
  theta_hat/1 -> Cos1/1, Cos/1
  Cos/1 -> Gain3/1, Product1/2
  Gain/1 -> Vector Concatenate4/3
  omega_hat/1 -> Gain2/1, Gain1/1
  Gain2/1 -> Product/1
  Gain1/1 -> Product1/1
  Product1/1 -> Vector Concatenate4/4
  Constant3/1 -> Vector Concatenate1/1
  Constant2/1 -> Vector Concatenate1/2
  Gain3/1 -> Vector Concatenate1/3
  Product/1 -> Vector Concatenate1/4
  Matrix Concatenate/1 -> F/1
  Constant5/1 -> Reshape1/1
  Constant4/1 -> Reshape2/1
  Reshape2/1 -> Matrix Concatenate/3
  Reshape1/1 -> Matrix Concatenate/4
  Cos1/1 -> Gain/1, Product/2

== system mcb_pmsm_foc_sensorless_f28379d/Current Control/Input Scaling/Calculate position and speed/EKF Observer/EKF/K ==
  P_pre : Inport
  H : Inport  Port=2
  R : Inport  Port=3
  Add : Sum
  Divide : Product  Inputs=*/  Multiplication=Matrix(*)
  Matrix Multiply : Product  Multiplication=Matrix(*)
  Matrix Multiply1 : Product  Multiplication=Matrix(*)
  Scope : Scope
  Transpose : Math  Operator=transpose  SignedPower=on
  K : Outport
  wires:
  R/1 -> Add/2
  H/1 -> Matrix Multiply1/1, Transpose/1
  P_pre/1 -> Matrix Multiply/1
  Transpose/1 -> Matrix Multiply/2
  Matrix Multiply1/1 -> Add/1
  Divide/1 -> K/1
  Matrix Multiply/1 -> Divide/1, Matrix Multiply1/2
  Add/1 -> Scope/1, Divide/2

== system mcb_pmsm_foc_sensorless_f28379d/Current Control/Input Scaling/Calculate position and speed/EKF Observer/EKF/P ==
  K : Inport
  H : Inport  Port=2
  P_pre : Inport  Port=3
  I : Inport  Port=4
  Add : Sum  Inputs=+-
  Matrix Multiply : Product  Multiplication=Matrix(*)
  Matrix Multiply1 : Product  Multiplication=Matrix(*)
  P : Outport
  wires:
  I/1 -> Add/1
  K/1 -> Matrix Multiply1/1
  H/1 -> Matrix Multiply1/2
  Matrix Multiply1/1 -> Add/2
  Add/1 -> Matrix Multiply/1
  P_pre/1 -> Matrix Multiply/2
  Matrix Multiply/1 -> P/1

== system mcb_pmsm_foc_sensorless_f28379d/Current Control/Input Scaling/Calculate position and speed/EKF Observer/EKF/P_pre ==
  A : Inport
  P : Inport  Port=2
  Q : Inport  Port=3
  Add : Sum
  Matrix Multiply : Product  Multiplication=Matrix(*)
  Matrix Multiply1 : Product  Multiplication=Matrix(*)
  Transpose : Math  Operator=transpose  SignedPower=on
  P_pre : Outport
  wires:
  A/1 -> Transpose/1, Matrix Multiply/1
  P/1 -> Matrix Multiply/2
  Add/1 -> P_pre/1
  Q/1 -> Add/2
  Matrix Multiply1/1 -> Add/1
  Matrix Multiply/1 -> Matrix Multiply1/1
  Transpose/1 -> Matrix Multiply1/2

== system mcb_pmsm_foc_sensorless_f28379d/Current Control/Input Scaling/Calculate position and speed/EKF Observer/EKF/X_hat ==
  X_pre : Inport
  K : Inport  Port=2
  Z : Inport  Port=3
  H : Inport  Port=4
  Add : Sum
  Add1 : Sum  Inputs=+-
  Matrix Multiply : Product  Multiplication=Matrix(*)
  Matrix Multiply1 : Product  Multiplication=Matrix(*)
  X_hat : Outport
  wires:
  X_pre/1 -> Matrix Multiply1/2, Add/1
  K/1 -> Matrix Multiply/1
  Z/1 -> Add1/1
  H/1 -> Matrix Multiply1/1
  Matrix Multiply1/1 -> Add1/2
  Add1/1 -> Matrix Multiply/2
  Matrix Multiply/1 -> Add/2
  Add/1 -> X_hat/1

== system mcb_pmsm_foc_sensorless_f28379d/Current Control/Input Scaling/Calculate position and speed/EKF Observer/EKF/X_pre ==
  f : Inport
  X_hat : Inport  Port=2
  B : Inport  Port=3
  U : Inport  Port=4
  Add1 : Sum  OutMin=[0.001]  OutMax=[100]  AccumDataTypeStr=double
  Add2 : Sum  OutMin=[0.001]  OutMax=[100]  AccumDataTypeStr=double
  Gain : Gain  Gain=T
  Matrix Multiply1 : Product  Multiplication=Matrix(*)
  X_pre : Outport
  wires:
  B/1 -> Matrix Multiply1/1
  U/1 -> Matrix Multiply1/2
  X_hat/1 -> Add1/1
  Matrix Multiply1/1 -> Add2/2
  f/1 -> Add2/1
  Add2/1 -> Gain/1
  Gain/1 -> Add1/2
  Add1/1 -> X_pre/1

== system mcb_pmsm_foc_sensorless_f28379d/Current Control/Input Scaling/Calculate position and speed/EKF Observer/EKF/Z ==
  H : Inport
  X : Inport  Port=2
  Matrix Multiply : Product  Multiplication=Matrix(*)
  P_pre : Outport
  wires:
  H/1 -> Matrix Multiply/1
  Matrix Multiply/1 -> P_pre/1
  X/1 -> Matrix Multiply/2

== system mcb_pmsm_foc_sensorless_f28379d/Current Control/Input Scaling/Calculate position and speed/EKF Observer/EKF/f(G(x)) ==
  i_alpha : Inport
  i_beta : Inport  Port=2
  omega_hat : Inport  Port=3
  theta_hat : Inport  Port=4
  Add : Sum
  Add1 : Sum
  Constant : Constant  Value=0
  Cos : Trigonometry  Operator=cos
  Cos1 : Trigonometry
  Gain : Gain  Gain=-pmsm.Rs/pmsm.Ls
  Gain1 : Gain  Gain=pmsm.FluxPM/pmsm.Ld
  Gain2 : Gain  Gain=-pmsm.Rs/pmsm.Ls
  Gain3 : Gain  Gain=-pmsm.FluxPM/pmsm.Ld
  Product1 : Product
  Product2 : Product
  Vector Concatenate4 : Concatenate  NumInputs=4  Mode=Multidimensional array
  f : Outport
  wires:
  theta_hat/1 -> Cos/1, Cos1/1
  Gain1/1 -> Product1/1
  i_alpha/1 -> Gain/1
  Gain/1 -> Add/1
  omega_hat/1 -> Gain3/1, Vector Concatenate4/4, Gain1/1
  Cos1/1 -> Product1/2
  Product1/1 -> Add/2
  Add/1 -> Vector Concatenate4/1
  Vector Concatenate4/1 -> f/1
  i_beta/1 -> Gain2/1
  Gain2/1 -> Add1/1
  Gain3/1 -> Product2/1
  Cos/1 -> Product2/2
  Product2/1 -> Add1/2
  Add1/1 -> Vector Concatenate4/2
  Constant/1 -> Vector Concatenate4/3

== system mcb_pmsm_foc_sensorless_f28379d/Current Control/Input Scaling/Calculate position and speed/HFI/位置和转速观测器/两相静止坐标系提取高频信号 ==
  i_alpha : Inport
  i_beta : Inport  Port=2
  Delay : Delay  DelayLength=1
  Delay1 : Delay  DelayLength=1
  Gain : Gain  Gain=1/2
  Gain1 : Gain  Gain=1/2
  Sum2 : Sum  Inputs=|+-
  Sum3 : Sum  Inputs=|+-
  i_alpha_h : Outport  VectorParamsAs1DForOutWhenUnconnected=off
  i_beta_h : Outport  Port=2  VectorParamsAs1DForOutWhenUnconnected=off
  wires:
  i_alpha/1 -> Sum2/2, Delay/1
  Sum2/1 -> Gain/1
  Gain/1 -> i_alpha_h/1
  Gain1/1 -> i_beta_h/1
  i_beta/1 -> Sum3/2, Delay1/1
  Sum3/1 -> Gain1/1
  Delay1/1 -> Sum3/1
  Delay/1 -> Sum2/1
